simulink model "bangBangD"  (R2017b)
settings: Solver=FixedStepAuto  StartTime=0.0  StopTime=1  FixedStep=0.025  RelTol=1e-3  EnableMultiTasking=on
values from neighbouring files (symbols this model uses):
  tF = yF(end)    [p1d.m]
settings Model: Creator=Soutrik  LastModifiedBy=Soutrik

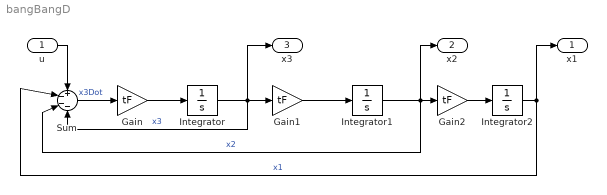
== system bangBangD ==
  u : Inport
  Gain : Gain  Gain=tF
  Gain1 : Gain  Gain=tF
  Gain2 : Gain  Gain=tF
  Integrator : Integrator  InitialCondition=1
  Integrator1 : Integrator  InitialCondition=1
  Integrator2 : Integrator  InitialCondition=1
  Sum : Sum  Inputs=+---
  x1 : Outport
  x2 : Outport  Port=2
  x3 : Outport  Port=3
  wires:
  Integrator/1 -> x3/1, Sum/4, Gain1/1  "x3"
  Integrator1/1 -> x2/1, Sum/3, Gain2/1  "x2"
  Sum/1 -> Gain/1  "x3Dot"
  u/1 -> Sum/1
  Integrator2/1 -> Sum/2, x1/1  "x1"
  Gain/1 -> Integrator/1
  Gain1/1 -> Integrator1/1
  Gain2/1 -> Integrator2/1
